simulink model "controller_angular_rate_yaw"  (R2021a)
settings: Solver=FixedStepAuto  StartTime=0.0  StopTime=10.0  FixedStep=0.002  RelTol=1e-3
undefined symbols (not defined in the file): body_rates_dterm_cutoff, body_rates_filter_denom, body_rates_filter_num, DiscIntNeverNeededParam, G_YR_OL_DENOM, G_YR_OL_NUM, K_rd, K_ri, K_rp, r_int_lim, r_max
libraries: simulink x1, pid_lib x1
settings Model: Creator=francois  LastModifiedBy=esl
settings SolverCC: AlgebraicLoopSolver=TrustRegion
settings DebuggingCC: SFMachineParentedDataDiag=warning

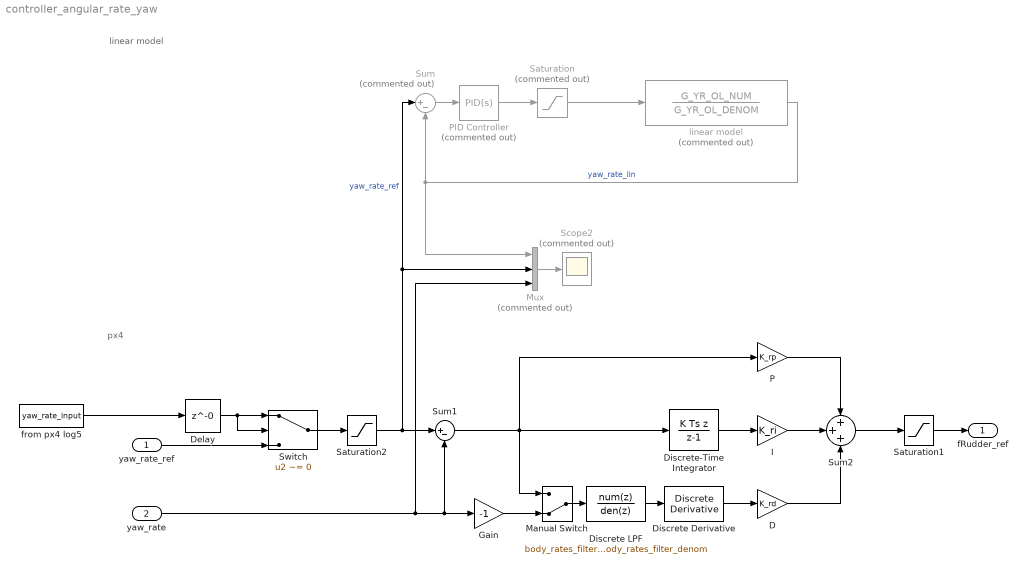
== system controller_angular_rate_yaw ==
  note: px4
  note: linear model
  yaw_rate_ref : Inport
  yaw_rate : Inport  Port=2
  D : Gain  Gain=K_rd
  Delay : Delay  DelayLength=0
  Discrete Derivative : simulink/Discrete/Discrete Derivative  gainval=1.0  ICPrevScaledInput=0.0  OutMin=[]  OutMax=[]  OutDataType=fixdt(1, 16)  OutScaling=2^-10  DoSatur=off
  Discrete LPF : DiscreteTransferFcn  Numerator=body_rates_filter_num  Denominator=body_rates_filter_denom
  Discrete-Time Integrator : DiscreteIntegrator  IntegratorMethod=Integration: Backward Euler  SampleTime=-1  LimitOutput=on  UpperSaturationLimit=r_int_lim  LowerSaturationLimit=-r_int_lim  ICPrevOutput=DiscIntNeverNeededParam  ICPrevScaledInput=DiscIntNeverNeededParam
  Gain : Gain  Gain=-1
  I : Gain  Gain=K_ri
  Manual Switch : ManualSwitch  CurrentSetting=0
  Mux : Mux  Commented=on  Inputs=3
  P : Gain  Gain=K_rp
  "PID Controller " : pid_lib/PID Controller  Commented=on  Controller=PID  Form=Parallel  TimeDomain=Continuous-time  UseExternalTs=off  SampleTime=-1  IntegratorMethod=Forward Euler  FilterMethod=Forward Euler  ControllerParametersSource=internal  P=K_rp  I=K_ri  D=K_rd  UseFilter=on  N=body_rates_dterm_cutoff*10  TunerSelectOption=Transfer Function Based (PID Tuner App)  InitialConditionSource=internal  InitialConditionForIntegrator=0  InitialConditionForFilter=0  DifferentiatorICPrevScaledInput=0  ExternalReset=none  TrackingMode=off  Kt=1  LimitOutput=off  SatLimitsSource=internal  UpperSaturationLimit=inf  LowerSaturationLimit=-inf  LinearizeAsGain=on  AntiWindupMode=none  Kb=1  POutMin=[]  POutMax=[]  IOutMin=[]  IOutMax=[]  DOutMin=[]  DOutMax=[]  NOutMin=[]  NOutMax=[]  SumOutMin=[]  SumOutMax=[]  SaturationOutMin=[]  SaturationOutMax=[]  PParamMin=[]  PParamMax=[]  IParamMin=[]  IParamMax=[]  DParamMin=[]  DParamMax=[]  NParamMin=[]  NParamMax=[]  KbParamMin=[]  KbParamMax=[]  KtParamMin=[]  KtParamMax=[]  KbOutMin=[]  KbOutMax=[]  KtOutMin=[]  KtOutMax=[]  IntegratorOutMin=[]  IntegratorOutMax=[]  FilterOutMin=[]  FilterOutMax=[]  SumI1OutMin=[]  SumI1OutMax=[]  SumI2OutMin=[]  SumI2OutMax=[]  SumI3OutMin=[]  SumI3OutMax=[]  SumI4OutMin=[]  SumI4OutMax=[]  SumDOutMin=[]  SumDOutMax=[]  DifferentiatorOutMin=[]  DifferentiatorOutMax=[]  FilterDiffOutCoefMin=[]  FilterDiffOutCoefMax=[]  ReciprocalOutMin=[]  ReciprocalOutMax=[]  SumDenOutMin=[]  SumDenOutMax=[]  SumNumOutMin=[]  SumNumOutMax=[]  DivideOutMin=[]  DivideOutMax=[]  UdiffTsProdOutMin=[]  UdiffTsProdOutMax=[]  NTsProdOutMin=[]  NTsProdOutMax=[]  UintegralTsProdOutMin=[]  UintegralTsProdOutMax=[]  UngainTsProdOutMin=[]  UngainTsProdOutMax=[]  IntegratorContinuousStateAttributes=''  IntegratorStateMustResolveToSignalObject=off  IntegratorRTWStateStorageClass=Auto  FilterContinuousStateAttributes=''  FilterStateMustResolveToSignalObject=off  FilterRTWStateStorageClass=Auto  ParallelPVariant=InternalParameters  IdealPVariant=Disabled  IVariant=InternalParameters  DVariant=InternalParameters  IntegratorVariant=Continuous  SatVariant=Disabled  AWVariant=Passthrough  PCopyVariant=Disabled  TRVariant=Disabled  FdbkBlocksVariant=Forward  IdealPFdbkVariant=Disabled  SatFdbkVariant=Disabled  DerivativeFilterVariant=ContFilter  NVariant=InternalParameters  NCopyVariant=Disabled  FilterICVariant=InternalICsFilter  IntegratorICVariant=InternalICs  ExternalResetVariant=Disabled  TRSumVariant=Passthrough  SumFdbkVariant=Disabled  SumVariant=Sum_PID  TsampFilterVariant=InternalTs  TsampNgainVariant=Passthrough  TsampIntegralVariant=Passthrough  ExternalSaturationOutDataTypeStr=Inherit: Same as second input
  Saturation : Saturate  Commented=on  UpperLimit=1  LowerLimit=-1
  Saturation1 : Saturate  UpperLimit=1  LowerLimit=-1
  Saturation2 : Saturate  UpperLimit=r_max  LowerLimit=-r_max
  Scope2 : Scope  Commented=on
  Sum : Sum  Commented=on  Inputs=|+-
  Sum1 : Sum  Inputs=|+-
  Sum2 : Sum  Inputs=+++
  Switch : Switch  Criteria=u2 ~= 0
  from px4 log5 : FromWorkspace  VariableName=yaw_rate_input
  linear model : TransferFcn  Commented=on  Numerator=G_YR_OL_NUM  Denominator=G_YR_OL_DENOM
  fRudder_ref : Outport
  wires:
  Sum/1 -> "PID Controller "/1
  yaw_rate_ref/1 -> Switch/3
  linear model/1 -> Mux/1, Sum/2  "yaw_rate_lin"
  Saturation/1 -> linear model/1
  "PID Controller "/1 -> Saturation/1
  Sum1/1 -> Discrete-Time Integrator/1, P/1, Manual Switch/1
  I/1 -> Sum2/2
  P/1 -> Sum2/1
  D/1 -> Sum2/3
  Discrete-Time Integrator/1 -> I/1
  Discrete Derivative/1 -> D/1
  Manual Switch/1 -> Discrete LPF/1
  Discrete LPF/1 -> Discrete Derivative/1
  Sum2/1 -> Saturation1/1
  Saturation1/1 -> fRudder_ref/1
  yaw_rate/1 -> Mux/3, Sum1/2, Gain/1
  Gain/1 -> Manual Switch/2
  Saturation2/1 -> Sum1/1, Sum/1, Mux/2  "yaw_rate_ref"
  Switch/1 -> Saturation2/1
  Delay/1 -> Switch/2, Switch/1
  from px4 log5/1 -> Delay/1
  Mux/1 -> Scope2/1
